simulink model "AutonomousModel_V5"  (R2020b)
settings: Solver=ode23t  StartTime=0.0  StopTime=180.1  FixedStep=0.05  RelTol=1e-3  EnableMultiTasking=on
model workspace (MAT data in the model file):
  DROP_VACCINE_TIME = 0.25
  GRID_SIDE = 0.457142857143
  HALF_TICKS_TO_DIST = 0.00174532925
  LATCHER_OFFSET = 0.3934603175
  LATCH_CELL_TIME = 0.5
  LOWER_PLATFORM_TIME = 0.5
  NUM_SURVEY_GRIDS = 7
  SPACE_SIDE = 0.152380952381
  SURVEY_GRIDS_CELLS = Simulink.Signal
  SURVEY_GRIDS_CELLS.DataType = 'double'
  SURVEY_GRIDS_CELLS.Dimensions = [1 7]
  SURVEY_GRIDS_CELLS.DimensionsMode = 'Fixed'
  SURVEY_GRIDS_CELLS.Complexity = 'real'
  SURVEY_GRIDS_CELLS.SampleTime = -1
  SURVEY_GRIDS_CELLS.SamplingMode = 'auto'
  SURVEY_GRIDS_CELLS.InitialValue = '[3 3 3 3 3 3 3]'
  SURVEY_GRIDS_COORDS = [5  6; 5  5; 5  4; 4  3; 5  2; 5  1; 6  0]
  SURVEY_TURN_ANGLE = 22.7856177106
  WAIT_CONFIRM_CELL_TIME = 0.08
  currentSurveyGridIndex = Simulink.Signal
  currentSurveyGridIndex.DataType = 'double'
  currentSurveyGridIndex.Dimensions = 1
  currentSurveyGridIndex.DimensionsMode = 'Fixed'
  currentSurveyGridIndex.Complexity = 'real'
  currentSurveyGridIndex.SampleTime = -1
  currentSurveyGridIndex.SamplingMode = 'auto'
  currentSurveyGridIndex.InitialValue = '0'
  fullRobotAngle = Simulink.Signal
  fullRobotAngle.DataType = 'double'
  fullRobotAngle.Dimensions = 1
  fullRobotAngle.DimensionsMode = 'Fixed'
  fullRobotAngle.Complexity = 'real'
  fullRobotAngle.SampleTime = -1
  fullRobotAngle.SamplingMode = 'auto'
  fullRobotAngle.InitialValue = '0'
  mapForSim.obsMap = [0 0 0 0 0 0 0 0 0 0 0 0 ... (4194304 elements, 2048x2048)]
  mapForSim.scaleFactor = 409.6
  mapForSim.simMap = robotics.BinaryOccupancyGrid
  mapForSim.simMap.Grid = [1 1 1 1 1 1 1 1 1 1 1 1 ... (4194304 elements, 2048x2048)]
  mapForSim.simMap.LayerName = "binaryLayer"
  mapForSim.simMap.Index = matlabshared.autonomous.internal.CircularBufferIndex
  mapForSim.simMap.Index.Head = [1 1]
  mapForSim.simMap.Index.Size = [2048 2048]
  mapForSim.simMap.Index.NewRegions = [0 0 0 0]
  mapForSim.simMap.Index.DropEntireMap = 0
  mapForSim.simMap.Index.DropTwoRegions = [0 0]
  mapForSim.simMap.Buffer = matlabshared.autonomous.internal.CircularBuffer
  mapForSim.simMap.Buffer.ConstVal = 0
  mapForSim.simMap.Buffer.DataType = 'logical'
  mapForSim.simMap.Buffer.Index = matlabshared.autonomous.internal.CircularBufferIndex
  mapForSim.simMap.Buffer.Index.Head = [1 1]
  mapForSim.simMap.Buffer.Index.Size = [2048 2048]
  mapForSim.simMap.Buffer.Index.NewRegions = [0 0 0 0]
  mapForSim.simMap.Buffer.Index.DropEntireMap = 0
  mapForSim.simMap.Buffer.Index.DropTwoRegions = [0 0]
  mapForSim.simMap.Buffer.Buffer = [1 1 1 1 1 1 1 1 1 1 1 1 ... (4194304 elements, 2048x2048)]
  mapForSim.simMap.DefaultValueInternal = 0
  mapForSim.simMap.HasParent = 0
  mapForSim.simMap.Resolution = 409.6
  mapForSim.simMap.GridSize = [2048 2048]
  mapForSim.simMap.GridOriginInLocal = [0 0]
  mapForSim.simMap.LocalOriginInWorld = [0 0]
  mapForSim.simMap.Width = 5
  mapForSim.simMap.Height = 5
  mapForSim.simMap.LocalOriginInWorldInternal = [0 0]
  moveDir = Simulink.Signal
  moveDir.DataType = 'double'
  moveDir.Dimensions = 1
  moveDir.DimensionsMode = 'Fixed'
  moveDir.Complexity = 'real'
  moveDir.SampleTime = -1
  moveDir.SamplingMode = 'auto'
  moveDir.InitialValue = '0'
  occGrid = robotics.BinaryOccupancyGrid
  occGrid.Grid = [1 1 1 1 1 1 1 1 1 1 1 1 ... (4194304 elements, 2048x2048)]
  occGrid.LayerName = "binaryLayer"
  occGrid.Index = matlabshared.autonomous.internal.CircularBufferIndex
  occGrid.Index.Head = [1 1]
  occGrid.Index.Size = [2048 2048]
  occGrid.Index.NewRegions = [0 0 0 0]
  occGrid.Index.DropEntireMap = 0
  occGrid.Index.DropTwoRegions = [0 0]
  occGrid.Buffer = matlabshared.autonomous.internal.CircularBuffer
  occGrid.Buffer.ConstVal = 0
  occGrid.Buffer.DataType = 'logical'
  occGrid.Buffer.Index = matlabshared.autonomous.internal.CircularBufferIndex
  occGrid.Buffer.Index.Head = [1 1]
  occGrid.Buffer.Index.Size = [2048 2048]
  occGrid.Buffer.Index.NewRegions = [0 0 0 0]
  occGrid.Buffer.Index.DropEntireMap = 0
  occGrid.Buffer.Index.DropTwoRegions = [0 0]
  occGrid.Buffer.Buffer = [1 1 1 1 1 1 1 1 1 1 1 1 ... (4194304 elements, 2048x2048)]
  occGrid.DefaultValueInternal = 0
  occGrid.HasParent = 0
  occGrid.Resolution = 409.6
  occGrid.GridSize = [2048 2048]
  occGrid.GridOriginInLocal = [0 0]
  occGrid.LocalOriginInWorld = [0 0]
  occGrid.Width = 5
  occGrid.Height = 5
  occGrid.LocalOriginInWorldInternal = [0 0]
  oldDetectedCellType = Simulink.Signal
  oldDetectedCellType.DataType = 'double'
  oldDetectedCellType.Dimensions = 1
  oldDetectedCellType.DimensionsMode = 'Fixed'
  oldDetectedCellType.Complexity = 'real'
  oldDetectedCellType.SampleTime = -1
  oldDetectedCellType.SamplingMode = 'auto'
  oldDetectedCellType.InitialValue = 'nan'
  onlyTrackUninfectedCells = Simulink.Signal
  onlyTrackUninfectedCells.DataType = 'boolean'
  onlyTrackUninfectedCells.Dimensions = 1
  onlyTrackUninfectedCells.DimensionsMode = 'Fixed'
  onlyTrackUninfectedCells.Complexity = 'real'
  onlyTrackUninfectedCells.SampleTime = -1
  onlyTrackUninfectedCells.SamplingMode = 'auto'
  onlyTrackUninfectedCells.InitialValue = 'false'
  prevLTicks = Simulink.Signal
  prevLTicks.DataType = 'double'
  prevLTicks.Dimensions = 1
  prevLTicks.DimensionsMode = 'Fixed'
  prevLTicks.Complexity = 'real'
  prevLTicks.SampleTime = -1
  prevLTicks.SamplingMode = 'auto'
  prevLTicks.InitialValue = '0'
  prevRTicks = Simulink.Signal
  prevRTicks.DataType = 'double'
  prevRTicks.Dimensions = 1
  prevRTicks.DimensionsMode = 'Fixed'
  prevRTicks.Complexity = 'real'
  prevRTicks.SampleTime = -1
  prevRTicks.SamplingMode = 'auto'
  prevRTicks.InitialValue = '0'
  straightDistTraveled = Simulink.Signal
  straightDistTraveled.DataType = 'double'
  straightDistTraveled.Dimensions = 1
  straightDistTraveled.DimensionsMode = 'Fixed'
  straightDistTraveled.Complexity = 'real'
  straightDistTraveled.SampleTime = -1
  straightDistTraveled.SamplingMode = 'auto'
  straightDistTraveled.InitialValue = '0'
  unsavedUninfectedCells = Simulink.Signal
  unsavedUninfectedCells.DataType = 'double'
  unsavedUninfectedCells.Dimensions = 1
  unsavedUninfectedCells.DimensionsMode = 'Fixed'
  unsavedUninfectedCells.Complexity = 'real'
  unsavedUninfectedCells.SampleTime = -1
  unsavedUninfectedCells.SamplingMode = 'auto'
  unsavedUninfectedCells.InitialValue = '12'
  xPos = Simulink.Signal
  xPos.DataType = 'double'
  xPos.Dimensions = 1
  xPos.DimensionsMode = 'Fixed'
  xPos.Complexity = 'real'
  xPos.SampleTime = -1
  xPos.SamplingMode = 'auto'
  xPos.InitialValue = '-0.4071428571'
  yPos = Simulink.Signal
  yPos.DataType = 'double'
  yPos.Dimensions = 1
  yPos.DimensionsMode = 'Fixed'
  yPos.Complexity = 'real'
  yPos.SampleTime = -1
  yPos.SamplingMode = 'auto'
  yPos.InitialValue = '1.6'
undefined symbols (not defined in the file): cellLevel, cellPose, cellTypeArray, FloorSurface, isoPoses, platformPoses, PlowSurface, Ref, RobotSurface, WallSurface, X, Y, Z
libraries: sm_lib x286, nesl_utility x157, simulink x72, pid_lib x3
(part 1 of 16)
settings Model: NumberOfSteps=1000  EnablePacing=on  PacingRate=1000  ExtModeTrigDuration=25  OrderedModelArguments=off  Creator=scastro  LastModifiedBy=wanga
settings SolverCC: AlgebraicLoopSolver=LineSearch
settings DataIOCC: LimitDataPoints=on  SignalLogging=off  ReturnWorkspaceOutputs=off
settings OptimizationCC: DefaultParameterBehavior=Inlined  PassReuseOutputArgsAs=Individual arguments  MaxStackSize=64  EfficientTunableParamExpr=on
settings DebuggingCC: ReadBeforeWriteMsg=DisableAll  WriteAfterWriteMsg=DisableAll  WriteAfterReadMsg=DisableAll  MultiTaskDSMMsg=none  ParameterPrecisionLossMsg=none  ParameterTunabilityLossMsg=error  UnconnectedLineMsg=none  AllowSymbolicDim=off  SFUnexpectedBacktrackingDiag=warning  SFNoUnconditionalDefaultTransitionDiag=warning  SFExecutionAtInitializationDiag=none  ArithmeticOperatorsInVariantConditions=warning
settings HardwareCC: ProdBitPerPointer=32  ProdBitPerSizeT=32  ProdBitPerPtrDiffT=32  ProdLargestAtomicInteger=Long  ProdLargestAtomicFloat=Double  ProdWordSize=32  ProdHWDeviceType=ARM Compatible->ARM Cortex
settings ModelReferenceCC: UpdateModelReferenceTargets=IfOutOfDate
settings SFSimCC: SFSimEcho=off  SimUseLocalCustomCode=off  MATLABDynamicMemAlloc=off  CustomCodeUndefinedFunction=UseInterfaceOnly
settings RTWCC: Description=Embedded Coder  SystemTargetFile=ert.tlc  TemplateMakefile=ert_default_tmf  GenerateReport=on  RTWUseLocalCustomCode=off  Toolchain=GNU Tools for ARM Embedded Processors  IncludeHyperlinkInReport=on  LaunchReport=on  GenerateTraceInfo=on  GenerateTraceReport=on  GenerateTraceReportSl=on  GenerateTraceReportSf=on  GenerateTraceReportEml=on
settings CodeAppCC: ForceParamTrailComments=on  IgnoreCustomStorageClasses=off  OperatorAnnotations=on  SimulinkDataObjDesc=on  SFDataObjDesc=on  InsertBlockDesc=on
settings ERTTargetCC: ExtModeStaticAllocSize=2048  ERTCustomFileTemplate=example_file_process.tlc
settings ConfigComp: CovMetricSettings=dw  CovSaveCumulativeToWorkspaceVar=on  CovSaveSingleToWorkspaceVar=on  CovExternalEMLEnable=off  CovSFcnEnable=off
settings SimscapeCC: SimscapeNominalValues="[{\"value\":\"10\",\"unit\":\"V\"},{\"value\":\"1\",\"unit\":\"A\"},{\"value\":\"10\",\"unit\":\"N*m\"},{\"value\":\"10\",\"unit\":\"bar\"},{\"value\":\"100\",\"unit\":\"kJ/kg\"},{\"value\":\"1\",\"unit\":\"kW\"},{\"value\":\"300\",\"unit\":\"K\"},{\"value\":\"100\",\"unit\":\"cm^3/s\"},{\"value\":\"1\",\"unit\":\"kN\"},{\"value\":\"1\",\"unit\":\"g/cm^3\"},{\"value\":\"1\",\"unit\":\"l\"},{\"value\":\"1\",\"unit\":\"cm^2\"},{\"value\":\"60\",\"unit\":\"Hz\"}]"  SimscapeLogOpenViewer=on  SimscapeLogDataHistory=10000
settings ConfigurationSet: Description=SimMechanics 2G
settings DiagnosticsConfigSet: SimMechanicsRigidlyBoundBlock=none
settings ExplorerConfigSet: InternalSimMechanicsExplorerSettings="<ExplorerConfiguration><canonicalview>default</canonicalview><AnimationSetting><BasePlaybackSpeed>1.0</BasePlaybackSpeed><PlaybackSpeedFactor>1.0</PlaybackSpeedFactor></AnimationSetting><TilePanel><TileInfo><Tiles Columns=\"1\" Count=\"1\" Rows=\"1\"><Column Weight=\"1\"/><Row Weight=\"1\"/><Tile Height=\"1\" Width=\"1\" X=\"0\" Y=\"0\"/></Tiles></TileInfo><SceneInfo><SceneViewer><BGColor><R>0.60000002384185791</R><G>0.60000002384185791</G><B>0.60000002384185791</B></BGColor><Camera><DoPerspective>off</DoPerspective><Position><X>0.310056035483453618</X><Y>0.109095541278226044</Y><Z>4.98936036725367327</Z></Position><Center><X>0.310056035483453618</X><Y>0.109095541278226044</Y><Z>-0.0112921193492265814</Z></Center><Up><X>0</X><Y>1</Y><Z>-0</Z></Up><ViewLimDist>1</ViewLimDist><YLim>2.36524049999999963</YLim><XLim>2.81382059482758606</XLim></Camera></SceneViewer></SceneInfo></TilePanel><MechEditorPanel><Cameras><Camera><Id>Camera1</Id><Value><Name>RobotView</Name><NativeCamera><PositionTrackingFeature>BEST_Robotics_2020_Game_Double_Click.BEST_2020_Robot.Body.RobotCamera.F</PositionTrackingFeature><CenterTrackingFeature>BEST_Robotics_2020_Game_Double_Click.BEST_2020_Robot.Body.RobotCamera.F</CenterTrackingFeature><UpVectorTrackingFeature>BEST_Robotics_2020_Game_Double_Click.BEST_2020_Robot.Body.RobotCamera.F</UpVectorTrackingFeature><CenterTrackingOrigin>off</CenterTrackingOrigin><CenterTrackingDirection>+X</CenterTrackingDirection><UpVectorTrackingDirection>+Z</UpVectorTrackingDirection></NativeCamera></Value></Camera></Cameras><GfxPanelCameraMap/><VideoCreator><PlaybackSpeedRatio>1.0</PlaybackSpeedRatio><FrameRate>16</FrameRate><VideoFormat>Motion JPEG AVI</VideoFormat><FrameSize>auto</FrameSize></VideoCreator></MechEditorPanel></ExplorerConfiguration>"

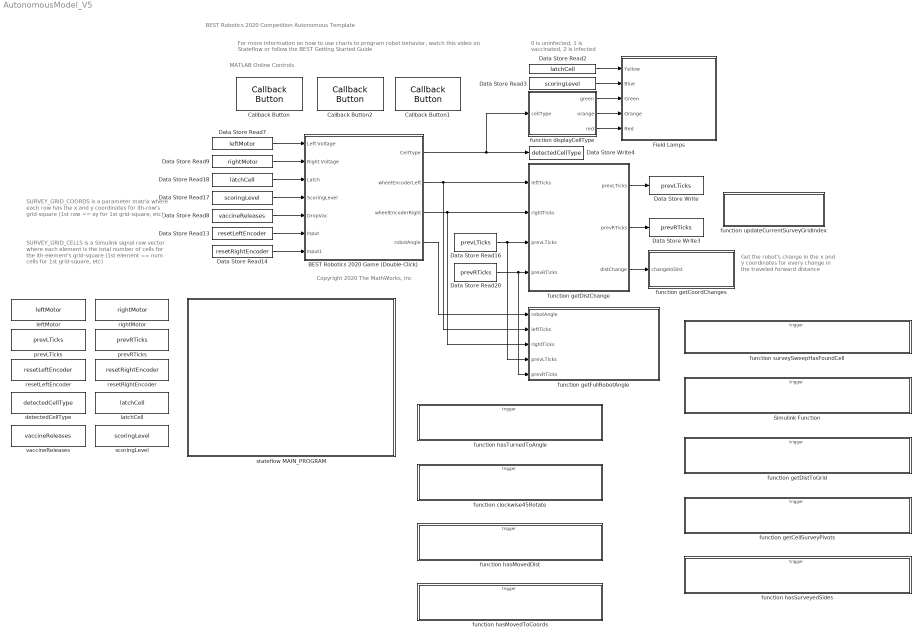
== system AutonomousModel_V5 ==
  note: 0 is uninfected, 1 is vaccinated, 2 is infected
  note: SURVEY_GRID_CELLS is a Simulink signal row vector where each element is the total number of cells for the ith-element's grid-square (1st element == num cells for 1st grid-square, etc)
  note: SURVEY_GRID_COORDS is a parameter matrix where each row has the x and y coordinates for ith-row's grid-square (1st row == xy for 1st grid-square, etc)
  note: MATLAB Online Controls
  note: For more information on how to use charts to program robot behavior,
      | watch this video on Stateflow or follow the BEST Getting Started Guide
  note: BEST Robotics 2020 Competition Autonomous Template
  note: Copyright 2020 The MathWorks, Inc
  note: Get the robot's change in the x and y coordinates for
      | every change in the traveled forward distance
  BEST Robotics 2020 Game (Double-Click) : Subsystem  mask(RP BEST Robotics 2020 Challenge){gameTime=180, field=Practice 2, rvis=off, sensor=off, autoField=on, wheelBase=0.5, wheelRadius=0.1, robotColor=[0.5 0 0], wheelThickness=0.025, chassisThickness=0.05, wheelMass=1, chassisMass=1.5}
      mask prompts: gameTime "Game Time (s)"; field "Field Layout"; rvis "Show cell type after run (Runs slower)"; sensor "Activate Gripper Sensor (Not allowed during competition)"; autoField "Autonomous Configuration"; wheelBase "Distance between wheels [m]"; wheelRadius "Wheel radius [m]"; robotColor "Color [R G B]"; wheelThickness "Wheel Thickness [m]"; chassisThickness "Chassis Thickness [m]"; wheelMass "Wheel Mass [kg]"; chassisMass "Chassis Mass [kg]"
      mask help:
      | This block contains a virtual game for the BEST Robotics 2020 competition. Please refere to the instructions provided by competition organizers for more information on game rules.
      |
      | Inputs:
      | Motor Voltages (Torque) [-127 to 127]
      | LatchCell (Pickup Cell) [0 or 1]
      | ScoringLevel (Floor or Platform) [0 or 1]
      | DropVac (Release vaccine) [0 or 1] Array of 3
      |
      | Outputs:
      | Cell Type (Uninfected, Immune, Infected) [0 ,1 or 2]
      | Sensors (See inside block for sensor properties and outputs)
      |
      | For MATLAB and Simulink related questions please email: roboticsarena@mathworks.com
      mask init:
      | autochoice=get_param(gcb,'autoField');
      | choice=get_param(gcb,'field');
      | time=get_param(gcb,'gameTime');
      | set_param(gcs,'StopTime',num2str(str2num(time)+0.1));
      | 
      | if strcmp(choice,'Practice 1')
      |   BEST2020GameConfig1 
      | elseif strcmp(choice,'Practice 2')
      |   BEST2020GameConfig2 
      | elseif strcmp(choice,'Practice 3')
      |   BEST2020GameConfig3 
      | elseif strcmp(choice,'Random')
      |   BEST2020GameConfigRand
      | elseif strcmp(autochoice,"on")
      |    if strcmp(choice,'Competition 1 (Provided during competition)')
      |      BEST2020GameConfigAuto1
      |    elseif strcmp(choice,'Competition 2 (Provided during competition)')
      |      BEST2020GameConfigAuto2
      |    elseif strcmp(choice,'Competition 3 (Provided during competition)')
      |      BEST2020GameConfigAuto3
      |    elseif strcmp(choice,'Competition 4 (Provided during competition)')
      |      BEST2020GameConfigAuto4
      |    elseif strcmp(choice,'Competition 5 (Provided during competition)')
      |      BEST2020GameConfigAuto5
      |    elseif strcmp(choice,'Competition 6 (Provided during competition)')
      |      BEST2020GameConfigAuto6
      |    elseif strcmp(choice,'Competition 7 (Provided during competition)')
      |      BEST2020GameConfigAuto7
      |    elseif strcmp(choice,'Competition 8 (Provided during competition)')
      |      BEST2020GameConfigAuto8
      |    else
      |      BEST2020GameConfigAuto1
      |    end
      | elseif strcmp(choice,'Competition 1 (Provided during competition)')
      |   BEST2020GameConfigComp1
      | elseif strcmp(choice,'Competition 2 (Provided during competition)')
      |   BEST2020GameConfigComp2
      | elseif strcmp(choice,'Competition 3 (Provided during competition)')
      |   BEST2020GameConfigComp3
      | elseif strcmp(choice,'Competition 4 (Provided during competition)')
      |   BEST2020GameConfigComp4
      | elseif strcmp(choice,'Competition 5 (Provided during competition)')
      |   BEST2020GameConfigComp5
      | elseif strcmp(choice,'Competition 6 (Provided during competition)')
      |   BEST2020GameConfigComp6
      | elseif strcmp(choice,'Competition 7 (Provided during competition)')
      |   BEST2020GameConfigComp7
      | elseif strcmp(choice,'Competition 8 (Provided during competition)')
      |   BEST2020GameConfigComp8
      | else
      |   BEST2020GameConfig1 
      | end
      mask TypeOptions field: Practice 1 | Practice 2 | Practice 3 | Random | Competition 1 (Provided during competition) | Competition 2 (Provided during competition) | Competition 3 (Provided during competition) | Competition 4 (Provided during competition) | Competition 5 (Provided during competition) | Competition 6 (Provided during competition) | Competition 7 (Provided during competition) | Competition 8 (Provided during competition)
      mask Callback rvis:
      | visual=get_param(gcb,'rvis');
      | for i=1:21
      |     if strcmp(visual,'off')
      |         set_param([gcb '/Cells/Object' num2str(i) '/EndVisuals'],'Commented','on');
      |     else
      |         set_param([gcb '/Cells/Object' num2str(i) '/EndVisuals'],'Commented','off');
      |     end
      | end
      mask TypeOptions wheelThickness: BEST 2020 Robot/wheelThickness
      mask TypeOptions chassisThickness: BEST 2020 Robot/chassisThickness
      mask TypeOptions wheelMass: BEST 2020 Robot/wheelMass
      mask TypeOptions chassisMass: BEST 2020 Robot/chassisMass
      mask DialogControl Container8 Prompt: Game Settings
      mask DialogControl Container4 Prompt: Robot settings
      mask Display:
      | image('BEST2020Environment.png')
      | port_label('input',1,'LeftMotor')
      | port_label('input',2,'RightMotor')
      | port_label('input',3,'LatchCell')
      | port_label('input',4,'ScoringLevel')
      | port_label('input',5,'DropVac')
      | port_label('output',1,'CellType')
      | port_label('output',2,'LeftEncoder')
      | port_label('output',3,'RightEncoder')
      | port_label('output',4,'RobotAngle')
  Callback Button : CallbackButton  ButtonText=Create Simulation Video (FPV)
      settings: ClickFcn=|
      | %% Simulate Model and Create Video
      | model=gcs;
      | disp(['Simulating Model: ' model '...'])
      | w=waitbar(0,['Simulating Model: ' model '...']);
      | set_param(model, 'EnablePacing', 'off');
      | sim(model);
      | set_param(model, 'EnablePacing', 'on');
      | disp('Creating Simulation Video...')
      | waitbar(0.5,w,'Creating Simulation Video...')
      | smwritevideo(model,model,'FrameRate',16,'FrameSize',[1280 720],'Tile',1)
      | disp('Animation window will close when completed')
      | waitbar(1,w,'Animation window will close when completed')
      | pause(5)
      | close(w)
  Callback Button1 : CallbackButton  ButtonText=Re-play Simulation Video
      settings: ClickFcn=|
      | %% Playback Simulation Video
      | disp('Replaying Simulation Video...')
      | videoReader = VideoReader([gcs '.avi']);
      | videoPlayer = vision.VideoPlayer('Position',[100 100 1280 720]);
      | 
      | % Play video. Every call to the step method reads another frame.
      | 
      | while hasFrame(videoReader)
      |    frame = readFrame(videoReader);
      |    step(videoPlayer,frame);
      |    pause(1/16);
      | end
      | disp('Done replaying simulation video')
  Callback Button2 : CallbackButton  ButtonText=Create Simulation Video (Top View)
      settings: ClickFcn=|
      | %% Simulate Model and Create Video
      | model=gcs;
      | disp(['Simulating Model: ' model '...'])
      | w=waitbar(0,['Simulating Model: ' model '...']);
      | set_param(model, 'EnablePacing', 'off');
      | sim(model);
      | set_param(model, 'EnablePacing', 'on');
      | disp('Creating Simulation Video...')
      | waitbar(0.5,w,'Creating Simulation Video...')
      | smwritevideo(model,model,'FrameRate',16,'FrameSize',[1280 720],'Tile',3)
      | disp('Animation window will close when completed')
      | waitbar(1,w,'Animation window will close when completed')
      | pause(5)
      | close(w)
  Data Store Read13 : DataStoreRead  DataStoreName=resetLeftEncoder
  Data Store Read14 : DataStoreRead  DataStoreName=resetRightEncoder
  Data Store Read16 : DataStoreRead  DataStoreName=prevLTicks
  Data Store Read17 : DataStoreRead  DataStoreName=scoringLevel
  Data Store Read18 : DataStoreRead  DataStoreName=latchCell
  Data Store Read2 : DataStoreRead  DataStoreName=latchCell
  Data Store Read20 : DataStoreRead  DataStoreName=prevRTicks
  Data Store Read3 : DataStoreRead  DataStoreName=scoringLevel
  Data Store Read7 : DataStoreRead  DataStoreName=leftMotor
  Data Store Read8 : DataStoreRead  DataStoreName=vaccineReleases
  Data Store Read9 : DataStoreRead  DataStoreName=rightMotor
  Data Store Write : DataStoreWrite  DataStoreName=prevLTicks
  Data Store Write3 : DataStoreWrite  DataStoreName=prevRTicks
  Data Store Write4 : DataStoreWrite  DataStoreName=detectedCellType
  Field Lamps : Subsystem
      mask Display:
      | image('lamps.PNG')
      | port_label('input',1,'Yellow')
      | port_label('input',2,'Blue')
      | port_label('input',3,'Green')
      | port_label('input',4,'Orange')
      | port_label('input',5,'Red')
  Simulink Function : Subsystem  TreatAsAtomicUnit=on
  detectedCellType : DataStoreMemory  DataStoreName=detectedCellType  ReadBeforeWriteMsg=warning  WriteAfterWriteMsg=warning  WriteAfterReadMsg=warning  ShowAdditionalParam=off  OutDataTypeStr=double  Dimensions=1
  function clockwise45Rotate : Subsystem  TreatAsAtomicUnit=on
  function displayCellType : MATLAB Function  TreatAsAtomicUnit=on
  function getCellSurveyPivots : Subsystem  TreatAsAtomicUnit=on
  function getCoordChanges : MATLAB Function  TreatAsAtomicUnit=on
  function getDistChange : MATLAB Function  TreatAsAtomicUnit=on
  function getDistToGrid : Subsystem  TreatAsAtomicUnit=on
  function getFullRobotAngle : MATLAB Function  TreatAsAtomicUnit=on
  function hasMovedDist : Subsystem  TreatAsAtomicUnit=on
  function hasMovedToCoords : Subsystem  TreatAsAtomicUnit=on
  function hasSurveyedSides : Subsystem  TreatAsAtomicUnit=on
  function hasTurnedToAngle : Subsystem  TreatAsAtomicUnit=on
  function surveySweepHasFoundCell : Subsystem  TreatAsAtomicUnit=on
  function updateCurrentSurveyGridIndex : MATLAB Function  TreatAsAtomicUnit=on
  latchCell : DataStoreMemory  DataStoreName=latchCell  ReadBeforeWriteMsg=warning  WriteAfterWriteMsg=warning  WriteAfterReadMsg=warning  ShowAdditionalParam=off  OutDataTypeStr=double  Dimensions=1
  leftMotor : DataStoreMemory  DataStoreName=leftMotor  ReadBeforeWriteMsg=warning  WriteAfterWriteMsg=warning  WriteAfterReadMsg=warning  ShowAdditionalParam=off  OutDataTypeStr=double  Dimensions=1
  prevLTicks : DataStoreMemory  DataStoreName=prevLTicks  ReadBeforeWriteMsg=warning  WriteAfterWriteMsg=warning  WriteAfterReadMsg=warning  ShowAdditionalParam=off  OutDataTypeStr=double  Dimensions=1
  prevRTicks : DataStoreMemory  DataStoreName=prevRTicks  ReadBeforeWriteMsg=warning  WriteAfterWriteMsg=warning  WriteAfterReadMsg=warning  ShowAdditionalParam=off  OutDataTypeStr=double  Dimensions=1
  resetLeftEncoder : DataStoreMemory  DataStoreName=resetLeftEncoder  ReadBeforeWriteMsg=warning  WriteAfterWriteMsg=warning  WriteAfterReadMsg=warning  ShowAdditionalParam=off  OutDataTypeStr=double  Dimensions=1
  resetRightEncoder : DataStoreMemory  DataStoreName=resetRightEncoder  ReadBeforeWriteMsg=warning  WriteAfterWriteMsg=warning  WriteAfterReadMsg=warning  ShowAdditionalParam=off  OutDataTypeStr=double  Dimensions=1
  rightMotor : DataStoreMemory  DataStoreName=rightMotor  ReadBeforeWriteMsg=warning  WriteAfterWriteMsg=warning  WriteAfterReadMsg=warning  ShowAdditionalParam=off  OutDataTypeStr=double  Dimensions=1
  scoringLevel : DataStoreMemory  DataStoreName=scoringLevel  ReadBeforeWriteMsg=warning  WriteAfterWriteMsg=warning  WriteAfterReadMsg=warning  ShowAdditionalParam=off  OutDataTypeStr=double  Dimensions=1
  stateflow MAIN_PROGRAM : Stateflow chart  TreatAsAtomicUnit=on
  vaccineReleases : DataStoreMemory  DataStoreName=vaccineReleases  ReadBeforeWriteMsg=warning  WriteAfterWriteMsg=warning  WriteAfterReadMsg=warning  InitialValue=[0 0 0]  VectorParams1D=off  ShowAdditionalParam=off  OutDataTypeStr=fixdt('double', 'DataTypeOverride', 'Off')  Dimensions=[1 3]
      settings: LockScale=on
  wires:
  Data Store Read9/1 -> BEST Robotics 2020 Game (Double-Click)/2(Right Voltage)
  BEST Robotics 2020 Game (Double-Click)/1(CellType) -> function displayCellType/1(cellType), Data Store Write4/1
  function displayCellType/1(green) -> Field Lamps/3(Green)
  function displayCellType/3(red) -> Field Lamps/5(Red)
  function displayCellType/2(orange) -> Field Lamps/4(Orange)
  Data Store Read8/1 -> BEST Robotics 2020 Game (Double-Click)/5(DropVac)
  Data Store Read7/1 -> BEST Robotics 2020 Game (Double-Click)/1(Left Voltage)
  Data Store Read13/1 -> BEST Robotics 2020 Game (Double-Click)/6(Input)
  Data Store Read14/1 -> BEST Robotics 2020 Game (Double-Click)/7(Input1)
  BEST Robotics 2020 Game (Double-Click)/3(wheelEncoderRight) -> function getFullRobotAngle/3(rightTicks), function getDistChange/2(rightTicks)
  Data Store Read20/1 -> function getFullRobotAngle/5(prevRTicks), function getDistChange/4("prevRTicks ")
  function getDistChange/3(distChange) -> function getCoordChanges/1(changeInDist)
  Data Store Read16/1 -> function getFullRobotAngle/4(prevLTicks), function getDistChange/3("prevLTicks ")
  BEST Robotics 2020 Game (Double-Click)/2(wheelEncoderLeft) -> function getFullRobotAngle/2(leftTicks), function getDistChange/1(leftTicks)
  BEST Robotics 2020 Game (Double-Click)/4(robotAngle) -> function getFullRobotAngle/1(robotAngle)
  Data Store Read17/1 -> BEST Robotics 2020 Game (Double-Click)/4(ScoringLevel)
  Data Store Read18/1 -> BEST Robotics 2020 Game (Double-Click)/3(Latch)
  Data Store Read3/1 -> Field Lamps/2(Blue)
  Data Store Read2/1 -> Field Lamps/1(Yellow)
  function getDistChange/1(prevLTicks) -> Data Store Write/1
  function getDistChange/2(prevRTicks) -> Data Store Write3/1

== system AutonomousModel_V5/BEST Robotics 2020 Game (Double-Click) ==
  note: DO NOT CHANGE THIS MODEL!
  Left Voltage : Inport
  Right Voltage : Inport  Port=2
  Latch : Inport  Port=3
  ScoringLevel : Inport  Port=4
  DropVac : Inport  Port=5
  Input : Inport  Port=6
  Input1 : Inport  Port=7
  Arena : Subsystem  mask(RP Grid Arena){length=7, width=7}
      mask prompts: length "Arena length [m]"; width "Arena width [m]"
      mask help: This block is an arena for robots to operate within. This arena implements contact between one robot and the walls and also introduces a floor grid for better visualization. Connect to other robots within the library using the corresponding "Robot" and "Ref" ports.
      mask DialogControl Container5 Prompt: Arena dimensions
      mask Display:
      | image('BEST2020Arena.png')
      | port_label('Lconn',1,'RP-Bus')
  BEST 2020 Robot : Subsystem  mask(RP Contact Tank Robot){robotId=1, wheelRadius=wheelRadius, wheelBase=wheelBase, wheelThickness=wheelThickness, chassisThickness=chassisThickness, startPose=[-2 0], choice=off, sensorTs=0.05, wheelMass=wheelMass, chassisMass=chassisMass, maxWheelTorque=2, wheelColor=[0.25 0.25 0.25], chassisColor=robotColor}
      mask prompts: robotId "Robot ID"; wheelRadius "Wheel Radius [m]"; wheelBase "Wheelbase [m]"; wheelThickness "Wheel Thickness [m]"; chassisThickness "Chassis Thickness [m]"; startPose "Start Position [m]"; choice "Reverse Start Position"; sensorTs "Sensor sample time [s]"; wheelMass "Wheel Mass [kg]"; chassisMass "Chassis Mass [kg]"; maxWheelTorque "Maximum wheel torque [N*m]"; wheelColor "Wheel Color"; chassisColor "Chassis Color"
      mask help:
      | This robot implements contact between the robot wheels and the floor of an arena. The stck-slip friction implemented using contact force libraries makes the robot behavior more realistic. The inputs to the robot are now motor torque, which is set using the Robotics Playground Motor blocks. The motor mappings are as follows:
      |
      | Motor 1 -> Left wheel motor torque
      | Motor 2 -> Right wheel motor torque
      mask DialogControl KinContainer Prompt: Kinematics
      mask DialogControl DynamicsContainer Prompt: Dynamics
      mask DialogControl AppearanceContainer Prompt: Appearance
      mask Display:
      | image('BEST2020Robot.png')
      | port_label('Rconn',1,'RP-Bus')
  Cells : Subsystem
      mask Display: image('BEST2020Cells.png')
  Compass Sensor : Subsystem  mask(RP Compass Sensor){sensorTs=.1}
      mask prompts: sensorTs "Sensor sample time [s]"
      mask help: This sensor outputs the rotation in degrees as measured from the robot center relative to the world coordinate frame.
      mask Help: web('compass_sensor.htm')
      mask DialogControl senCont Prompt: Sensor Characteristics
      mask Display:
      | color('white');
      | plot([100,100,100,100]*1,[100,100,100,100]*1);
      | plot([100,100,100,100]*0,[100,100,100,100]*0);
      | image('Compass.png','center')
      | color('blue');
  Game Control : Subsystem
  Left Encoder1 : Subsystem  mask(RP Motor Encoder){rstChoice=Reset by external signal, ticks=180, detectDir=on, sensorTs=.1}
      mask prompts: rstChoice "Reset option"; ticks "Ticks per rotation"; detectDir "Detect direction of rotation"; sensorTs "Sensor sample time [s]"
      mask help:
      | This block outputs the rotation in tick counts of an encoder conneted to the respective robot motor. You can set different sensor parameters from the mask or use the default settings.
      |
      | The most common use of motor encoders is to derive the position of an object. Start by converting the tick counts to revolutions of the motor shaft. You can later relate the revolutions of the motor shaft to more valuable robot information such as traveled distance by using robot dimensions like the wheel size.
      mask Help: web('encoder_sensor.htm')
      mask TypeOptions rstChoice: No reset | Reset by external signal
      mask DialogControl ParameterGroupVar Prompt: Settings
      mask Display:
      | color('white');
      | plot([100,100,100,100]*1,[100,100,100,100]*1);
      | plot([100,100,100,100]*0,[100,100,100,100]*0);
      | image('encoder.jpg','center')
  Right Encoder1 : Subsystem  mask(RP Motor Encoder){rstChoice=Reset by external signal, ticks=180, detectDir=on, sensorTs=.1}
      mask prompts: rstChoice "Reset option"; ticks "Ticks per rotation"; detectDir "Detect direction of rotation"; sensorTs "Sensor sample time [s]"
      mask help:
      | This block outputs the rotation in tick counts of an encoder conneted to the respective robot motor. You can set different sensor parameters from the mask or use the default settings.
      |
      | The most common use of motor encoders is to derive the position of an object. Start by converting the tick counts to revolutions of the motor shaft. You can later relate the revolutions of the motor shaft to more valuable robot information such as traveled distance by using robot dimensions like the wheel size.
      mask Help: web('encoder_sensor.htm')
      mask TypeOptions rstChoice: No reset | Reset by external signal
      mask DialogControl ParameterGroupVar Prompt: Settings
      mask Display:
      | color('white');
      | plot([100,100,100,100]*1,[100,100,100,100]*1);
      | plot([100,100,100,100]*0,[100,100,100,100]*0);
      | image('encoder.jpg','center')
  Vaccines : Subsystem
      mask Display: image('BEST2020Vaccines.png')
  CellType : Outport
  wheelEncoderLeft : Outport  Port=2
  wheelEncoderRight : Outport  Port=3
  robotAngle : Outport  Port=4
  wires:
  Right Voltage/1 -> BEST 2020 Robot/2(In2)
  Left Voltage/1 -> BEST 2020 Robot/1(In1)
  Latch/1 -> Cells/1(Latch)
  Cells/1(CellType) -> CellType/1
  Right Encoder1/1(Out1) -> wheelEncoderRight/1
  Left Encoder1/1(Out1) -> wheelEncoderLeft/1
  BEST 2020 Robot/3(angle) -> Compass Sensor/1(angle)
  Compass Sensor/1(Distance) -> robotAngle/1
  DropVac/1 -> Vaccines/2(Drop)
  ScoringLevel/1 -> Vaccines/1("ScoreLevel "), Cells/2(ScoringLevel)
  BEST 2020 Robot/1(leftMotorW) -> Left Encoder1/1(In1)
  BEST 2020 Robot/2(rightMotorW) -> Right Encoder1/1(In1)
  Input/1 -> Left Encoder1/2(Input)
  Input1/1 -> Right Encoder1/2(Input)
  connections:
  Vaccines/LConn1 -- Arena/LConn1 -- BEST 2020 Robot/RConn1 -- Cells/LConn1

== system AutonomousModel_V5/Field Lamps ==
  note: DO NOT EDIT
  note: Inputs should be 0 or 1
  Yellow : Inport
  Blue : Inport  Port=2
  Green : Inport  Port=3
  Orange : Inport  Port=4
  Red : Inport  Port=5
  tag scope: blueLamp=global, greenLamp=global, orangeLamp=global, redLamp=global, yellowLamp=global
  wires:
  Yellow/1 -> [yellowLamp]
  Blue/1 -> [blueLamp]
  Orange/1 -> [orangeLamp]
  Red/1 -> [redLamp]
  Green/1 -> [greenLamp]

== system AutonomousModel_V5/Simulink Function ==
  getNearestUnrescuedGrid : TriggerPort  TriggerType=function-call  IsSimulinkFunction=on  FunctionName=getNearestUnrescuedGrid  FunctionVisibility=scoped  VariantControl=(inherit)
  function getClosestValidGrid : MATLAB Function  TreatAsAtomicUnit=on
  rescueGridX : ArgOut  DisableCoverage=on  ArgumentName=rescueGridX
  rescueGridY : ArgOut  DisableCoverage=on  Port=2  ArgumentName=rescueGridY
  closestGridIndex : ArgOut  DisableCoverage=on  Port=3  ArgumentName=closestGridIndex
  wires:
  function getClosestValidGrid/1(closestGridX) -> rescueGridX/1
  function getClosestValidGrid/2(closestGridY) -> rescueGridY/1
  function getClosestValidGrid/3(closestGridIndex) -> closestGridIndex/1

== system AutonomousModel_V5/function clockwise45Rotate ==
  clockwise45Rotate : TriggerPort  TriggerType=function-call  IsSimulinkFunction=on  FunctionName=clockwise45Rotate  FunctionVisibility=scoped  VariantControl=(inherit)
  function clockwise45Rotate : MATLAB Function  TreatAsAtomicUnit=on
  oldX : ArgIn  DisableCoverage=on  ArgumentName=oldX
  oldY : ArgIn  Port=2  ArgumentName=oldY
  rotatedX : ArgOut  DisableCoverage=on  ArgumentName=rotatedX
  rotatedY : ArgOut  Port=2  ArgumentName=rotatedY
  wires:
  oldX/1 -> function clockwise45Rotate/1(oldX)
  oldY/1 -> function clockwise45Rotate/2(oldY)
  function clockwise45Rotate/1(rotatedX) -> rotatedX/1
  function clockwise45Rotate/2(rotatedY) -> rotatedY/1

== system AutonomousModel_V5/function getCellSurveyPivots ==
  getCellSurveyPivots : TriggerPort  TriggerType=function-call  IsSimulinkFunction=on  FunctionName=getCellSurveyPivots  FunctionVisibility=scoped  VariantControl=(inherit)
  function getCellSurveyCheckpoints : MATLAB Function  TreatAsAtomicUnit=on
  gridX : ArgIn  DisableCoverage=on  ArgumentName=gridX
  gridY : ArgIn  Port=2  ArgumentName=gridY
  pivotSide : ArgOut  DisableCoverage=on  PortDimensions=[1 1]  ArgumentName=pivotSide
  startPivotPoint : ArgOut  Port=2  PortDimensions=[1 2]  ArgumentName=startPivotPoint
  finalPoint : ArgOut  Port=3  PortDimensions=[1 2]  ArgumentName=finalPoint
  wires:
  gridX/1 -> function getCellSurveyCheckpoints/1(gridX)
  gridY/1 -> function getCellSurveyCheckpoints/2(gridY)
  function getCellSurveyCheckpoints/1(pivotSide) -> pivotSide/1
  function getCellSurveyCheckpoints/2(startPivotPoint) -> startPivotPoint/1
  function getCellSurveyCheckpoints/3(finalPoint) -> finalPoint/1

== system AutonomousModel_V5/function getDistToGrid ==
  getDistToGrid : TriggerPort  TriggerType=function-call  IsSimulinkFunction=on  FunctionName=getDistToGrid  FunctionVisibility=scoped  VariantControl=(inherit)
  MATLAB Function : MATLAB Function  TreatAsAtomicUnit=on
  gridX : ArgIn  DisableCoverage=on  ArgumentName=gridX
  gridY : ArgIn  DisableCoverage=on  Port=2  ArgumentName=gridY
  dist : ArgOut  DisableCoverage=on  ArgumentName=dist
  wires:
  MATLAB Function/1(dist) -> dist/1
  gridX/1 -> MATLAB Function/1(gridX)
  gridY/1 -> MATLAB Function/2(gridY)

== system AutonomousModel_V5/function hasMovedDist ==
  note: PID_SETTLE_TIME is measured in n*0.1 seconds,
      | meaning a value of 5 for this would mean a
      | requirement for the PID to turn the robot should
      | settle for 0.5 seconds before stopping
  hasMovedDist : TriggerPort  TriggerType=function-call  IsSimulinkFunction=on  FunctionName=hasMovedDist  FunctionVisibility=scoped  VariantControl=(inherit)
  Abs1 : Abs
  Data Store Memory2 : DataStoreMemory  DataStoreName=settledTime  ReadBeforeWriteMsg=warning  WriteAfterWriteMsg=warning  WriteAfterReadMsg=warning  ShowAdditionalParam=off  OutDataTypeStr=double  Dimensions=1
  Data Store Read6 : DataStoreRead  DataStoreName=settledTime
  Data Store Write1 : DataStoreWrite  DataStoreName=leftMotor
  Data Store Write2 : DataStoreWrite  DataStoreName=rightMotor
  GreaterThanOrEqual1 : RelationalOperator  OutDataTypeStr=boolean  RndMeth=Simplest
  PID Controller : pid_lib/PID Controller  Controller=P  Form=Parallel  TimeDomain=Discrete-time  UseExternalTs=on  SampleTime=0.1  IntegratorMethod=Forward Euler  FilterMethod=Forward Euler  ControllerParametersSource=internal  P=100  I=2  D=0.5  UseFilter=on  N=100  TunerSelectOption=Transfer Function Based (PID Tuner App)  InitialConditionSource=internal  InitialConditionForIntegrator=0  InitialConditionForFilter=0  DifferentiatorICPrevScaledInput=0  ExternalReset=none  TrackingMode=off  Kt=1  LimitOutput=on  SatLimitsSource=internal  UpperSaturationLimit=127  LowerSaturationLimit=-127  LinearizeAsGain=off  AntiWindupMode=none  Kb=1  RndMeth=Nearest  POutMin=[]  POutMax=[]  IOutMin=[]  IOutMax=[]  DOutMin=[]  DOutMax=[]  NOutMin=[]  NOutMax=[]  SumOutMin=[]  SumOutMax=[]  SaturationOutMin=[]  SaturationOutMax=[]  PParamMin=[]  PParamMax=[]  IParamMin=[]  IParamMax=[]  DParamMin=[]  DParamMax=[]  NParamMin=[]  NParamMax=[]  KbParamMin=[]  KbParamMax=[]  KtParamMin=[]  KtParamMax=[]  KbOutMin=[]  KbOutMax=[]  KtOutMin=[]  KtOutMax=[]  IntegratorOutMin=[]  IntegratorOutMax=[]  FilterOutMin=[]  FilterOutMax=[]  SumI1OutMin=[]  SumI1OutMax=[]  SumI2OutMin=[]  SumI2OutMax=[]  SumI3OutMin=[]  SumI3OutMax=[]  SumI4OutMin=[]  SumI4OutMax=[]  SumDOutMin=[]  SumDOutMax=[]  DifferentiatorOutMin=[]  DifferentiatorOutMax=[]  FilterDiffOutCoefMin=[]  FilterDiffOutCoefMax=[]  ReciprocalOutMin=[]  ReciprocalOutMax=[]  SumDenOutMin=[]  SumDenOutMax=[]  SumNumOutMin=[]  SumNumOutMax=[]  DivideOutMin=[]  DivideOutMax=[]  UdiffTsProdOutMin=[]  UdiffTsProdOutMax=[]  NTsProdOutMin=[]  NTsProdOutMax=[]  UintegralTsProdOutMin=[]  UintegralTsProdOutMax=[]  UngainTsProdOutMin=[]  UngainTsProdOutMax=[]  IntegratorContinuousStateAttributes=''  IntegratorStateMustResolveToSignalObject=off  IntegratorRTWStateStorageClass=Auto  FilterContinuousStateAttributes=''  FilterStateMustResolveToSignalObject=off  FilterRTWStateStorageClass=Auto  ParallelPVariant=InternalParameters  IdealPVariant=Disabled  IVariant=Disabled  DVariant=Disabled  IntegratorVariant=Disabled  SatVariant=Enabled  AWVariant=Disabled  PCopyVariant=Disabled  TRVariant=Disabled  FdbkBlocksVariant=Forward  IdealPFdbkVariant=Disabled  SatFdbkVariant=Disabled  DerivativeFilterVariant=Disabled  NVariant=Disabled  NCopyVariant=Disabled_SignalSpec  FilterICVariant=Disabled  IntegratorICVariant=Disabled  ExternalResetVariant=Disabled  TRSumVariant=Passthrough  SumFdbkVariant=Disabled  SumVariant=Passthrough_P  TsampFilterVariant=InternalTs  TsampNgainVariant=Passthrough  TsampIntegralVariant=Disabled  ExternalSaturationOutDataTypeStr=Inherit: Same as second input
  PID_DIST_TOLERANCE : Constant  Value=0.009
  PID_SETTLE_TIME : Constant  Value=2
  function getErrorDist : MATLAB Function  TreatAsAtomicUnit=on
  function getMoveDirSign : MATLAB Function  TreatAsAtomicUnit=on
  stateflow integrateSettleTime : Stateflow chart  TreatAsAtomicUnit=on
      settings: PortSchema="{\"entries\":[{\"content\":{\"sides\":[{\"content\":{\"connectorIds\":[\"In2\",\"In1\"]},\"type\":\"ConnectorPlacement.EquallySpacedRectSide\",\"uuid\":\"f923337d-3128-4ed8-bb4f-3ea7b5686e2d\"},{\"content\":{\"connectorIds\":[],\"side\":\"RIGHT\"},\"type\":\"ConnectorPlacement.EquallySpacedRectSide\",\"uuid\":\"39dc7172-a5aa-4f5c-b2a4-4c61f2fa72eb\"},{\"content\":{\"connectorIds\":[],\"side\":\"TOP\"},\"type\":\"ConnectorPlacement.EquallySpacedRectSide\",\"uuid\":\"39425eec-6ca1-4a0a-a982-d9b02b3e3e8f\"},{\"content\":{\"connectorIds\":[],\"side\":\"HIDDEN\"},\"type\":\"ConnectorPlacement.EquallySpacedRectSide\",\"uuid\":\"aee45ecb-1b8b-4c38-bfd6-fdbe8fac54d7\"}]},\"type\":\"ConnectorPlacement.EquallySpacedConnector\",\"uuid\":\"e05cbbda-f452-42ce-8e08-9c45c77a95c5\"}],\"packageUris\":[\"http://schema.mathworks.com/mf0/Connector/R2020b\"],\"version\":\"1.0\"}"
  stateflow postSettleDist : Stateflow chart  TreatAsAtomicUnit=on
  targetDist : ArgIn  DisableCoverage=on  ArgumentName=targetDist
  distHasSettled : ArgOut  DisableCoverage=on  OutDataTypeStr=boolean  ArgumentName=distHasSettled
  wires:
  GreaterThanOrEqual1/1 -> stateflow postSettleDist/1(distHasSettled), distHasSettled/1
  PID_SETTLE_TIME/1 -> GreaterThanOrEqual1/2
  PID_DIST_TOLERANCE/1 -> stateflow integrateSettleTime/1(TOLERANCE)
  Abs1/1 -> stateflow integrateSettleTime/2(error)
  Data Store Read6/1 -> GreaterThanOrEqual1/1
  function getErrorDist/1(errorDist) -> Abs1/1, PID Controller/1
  targetDist/1 -> function getErrorDist/1(targetDist)
  PID Controller/1 -> Data Store Write2/1, Data Store Write1/1, function getMoveDirSign/1(u)

== system AutonomousModel_V5/function hasMovedToCoords ==
  hasMovedToCoords : TriggerPort  TriggerType=function-call  IsSimulinkFunction=on  FunctionName=hasMovedToCoords  FunctionVisibility=scoped  VariantControl=(inherit)
  stateflow hasMovedToCoords : Stateflow chart  AncestorBlock=RoboticsPlayground/Utilities and Hardware/Stateflow  TreatAsAtomicUnit=on
  xCoord : ArgIn  DisableCoverage=on  ArgumentName=xCoord
  yCoord : ArgIn  Port=2  ArgumentName=yCoord
  useRobotPos : ArgIn  Port=3  ArgumentName=useRobotPos
  arrived : ArgOut  DisableCoverage=on  OutDataTypeStr=boolean  ArgumentName=arrived
  wires:
  xCoord/1 -> stateflow hasMovedToCoords/1(xCoord)
  yCoord/1 -> stateflow hasMovedToCoords/2(yCoord)
  stateflow hasMovedToCoords/1(hasArrived) -> arrived/1
  useRobotPos/1 -> stateflow hasMovedToCoords/3(useRobotPos)

== system AutonomousModel_V5/function hasSurveyedSides ==
  hasSurveyedSides : TriggerPort  TriggerType=function-call  IsSimulinkFunction=on  FunctionName=hasSurveyedSides  FunctionVisibility=scoped  VariantControl=(inherit)
  function getSurveyAngles : MATLAB Function  TreatAsAtomicUnit=on
  stateflow hasSurveyedSides : Stateflow chart  TreatAsAtomicUnit=on
  pivotSide : ArgIn  DisableCoverage=on  ArgumentName=pivotSide
  sidesSurveyed : ArgOut  DisableCoverage=on  OutDataTypeStr=boolean  ArgumentName=sidesSurveyed
  wires:
  function getSurveyAngles/3(returnAngle) -> stateflow hasSurveyedSides/3(returnAngle)
  stateflow hasSurveyedSides/1(hasSurveyedSides) -> sidesSurveyed/1
  function getSurveyAngles/2(secondSurveyAngle) -> stateflow hasSurveyedSides/2(secondSurveyAngle)
  pivotSide/1 -> function getSurveyAngles/1(pivotSide)
  function getSurveyAngles/1(firstSurveyAngle) -> stateflow hasSurveyedSides/1(firstSurveyAngle)

== system AutonomousModel_V5/function hasTurnedToAngle ==
  note: targetAngle should be from 0 to 360 degrees
  note: PID_SETTLE_TIME is measured in n*0.1 seconds,
      | meaning a value of 5 for this would mean a
      | requirement for the PID to turn the robot should
      | settle for 0.5 seconds before stopping
  hasTurnedToAngle : TriggerPort  TriggerType=function-call  IsSimulinkFunction=on  FunctionName=hasTurnedToAngle  FunctionVisibility=scoped  VariantControl=(inherit)
  Abs : Abs
  Data Store Memory2 : DataStoreMemory  DataStoreName=settledTime  ReadBeforeWriteMsg=warning  WriteAfterWriteMsg=warning  WriteAfterReadMsg=warning  ShowAdditionalParam=off  OutDataTypeStr=double  Dimensions=1
  Data Store Read2 : DataStoreRead  DataStoreName=settledTime
  Data Store Write4 : DataStoreWrite  DataStoreName=leftMotor
  Data Store Write5 : DataStoreWrite  DataStoreName=rightMotor
  Gain : Gain  Gain=-1
  GreaterThanOrEqual : RelationalOperator  OutDataTypeStr=boolean  RndMeth=Simplest
  PID Controller1 : pid_lib/PID Controller  Controller=PI  Form=Parallel  TimeDomain=Discrete-time  UseExternalTs=off  SampleTime=-1  IntegratorMethod=Forward Euler  FilterMethod=Forward Euler  ControllerParametersSource=internal  P=0.812779127376154  I=0  D=0  UseFilter=off  N=100  TunerSelectOption=Transfer Function Based (PID Tuner App)  InitialConditionSource=internal  InitialConditionForIntegrator=0.21807542656823095  InitialConditionForFilter=0  DifferentiatorICPrevScaledInput=0  ExternalReset=none  TrackingMode=off  Kt=1  LimitOutput=on  SatLimitsSource=internal  UpperSaturationLimit=127  LowerSaturationLimit=-127  LinearizeAsGain=off  AntiWindupMode=none  Kb=1  RndMeth=Nearest  POutMin=[]  POutMax=[]  IOutMin=[]  IOutMax=[]  DOutMin=[]  DOutMax=[]  NOutMin=[]  NOutMax=[]  SumOutMin=[]  SumOutMax=[]  SaturationOutMin=[]  SaturationOutMax=[]  PParamMin=[]  PParamMax=[]  IParamMin=[]  IParamMax=[]  DParamMin=[]  DParamMax=[]  NParamMin=[]  NParamMax=[]  KbParamMin=[]  KbParamMax=[]  KtParamMin=[]  KtParamMax=[]  KbOutMin=[]  KbOutMax=[]  KtOutMin=[]  KtOutMax=[]  IntegratorOutMin=[]  IntegratorOutMax=[]  FilterOutMin=[]  FilterOutMax=[]  SumI1OutMin=[]  SumI1OutMax=[]  SumI2OutMin=[]  SumI2OutMax=[]  SumI3OutMin=[]  SumI3OutMax=[]  SumI4OutMin=[]  SumI4OutMax=[]  SumDOutMin=[]  SumDOutMax=[]  DifferentiatorOutMin=[]  DifferentiatorOutMax=[]  FilterDiffOutCoefMin=[]  FilterDiffOutCoefMax=[]  ReciprocalOutMin=[]  ReciprocalOutMax=[]  SumDenOutMin=[]  SumDenOutMax=[]  SumNumOutMin=[]  SumNumOutMax=[]  DivideOutMin=[]  DivideOutMax=[]  UdiffTsProdOutMin=[]  UdiffTsProdOutMax=[]  NTsProdOutMin=[]  NTsProdOutMax=[]  UintegralTsProdOutMin=[]  UintegralTsProdOutMax=[]  UngainTsProdOutMin=[]  UngainTsProdOutMax=[]  IntegratorContinuousStateAttributes=''  IntegratorStateMustResolveToSignalObject=off  IntegratorRTWStateStorageClass=Auto  FilterContinuousStateAttributes=''  FilterStateMustResolveToSignalObject=off  FilterRTWStateStorageClass=Auto  ParallelPVariant=InternalParameters  IdealPVariant=Disabled  IVariant=InternalParameters  DVariant=Disabled  IntegratorVariant=Discrete  SatVariant=Enabled  AWVariant=Passthrough  PCopyVariant=Disabled  TRVariant=Disabled  FdbkBlocksVariant=Forward  IdealPFdbkVariant=Disabled  SatFdbkVariant=Disabled  DerivativeFilterVariant=Disabled  NVariant=Disabled  NCopyVariant=Disabled_SignalSpec  FilterICVariant=Disabled  IntegratorICVariant=InternalICs  ExternalResetVariant=Disabled  TRSumVariant=Passthrough  SumFdbkVariant=Disabled  SumVariant=Sum_PI  TsampFilterVariant=InternalTs  TsampNgainVariant=Passthrough  TsampIntegralVariant=Passthrough  ExternalSaturationOutDataTypeStr=Inherit: Same as second input
  PID Controller2 : pid_lib/PID Controller  Commented=on  Controller=PI  Form=Parallel  TimeDomain=Discrete-time  UseExternalTs=off  SampleTime=-1  IntegratorMethod=Forward Euler  FilterMethod=Forward Euler  ControllerParametersSource=internal  P=0.4220988064561398  I=245.15019805202533  D=0  UseFilter=off  N=100  TunerSelectOption=Transfer Function Based (PID Tuner App)  InitialConditionSource=internal  InitialConditionForIntegrator=0  InitialConditionForFilter=0  DifferentiatorICPrevScaledInput=0  ExternalReset=rising  TrackingMode=off  Kt=1  LimitOutput=on  SatLimitsSource=internal  UpperSaturationLimit=127  LowerSaturationLimit=-127  LinearizeAsGain=off  AntiWindupMode=none  Kb=1  RndMeth=Nearest  POutMin=[]  POutMax=[]  IOutMin=[]  IOutMax=[]  DOutMin=[]  DOutMax=[]  NOutMin=[]  NOutMax=[]  SumOutMin=[]  SumOutMax=[]  SaturationOutMin=[]  SaturationOutMax=[]  PParamMin=[]  PParamMax=[]  IParamMin=[]  IParamMax=[]  DParamMin=[]  DParamMax=[]  NParamMin=[]  NParamMax=[]  KbParamMin=[]  KbParamMax=[]  KtParamMin=[]  KtParamMax=[]  KbOutMin=[]  KbOutMax=[]  KtOutMin=[]  KtOutMax=[]  IntegratorOutMin=[]  IntegratorOutMax=[]  FilterOutMin=[]  FilterOutMax=[]  SumI1OutMin=[]  SumI1OutMax=[]  SumI2OutMin=[]  SumI2OutMax=[]  SumI3OutMin=[]  SumI3OutMax=[]  SumI4OutMin=[]  SumI4OutMax=[]  SumDOutMin=[]  SumDOutMax=[]  DifferentiatorOutMin=[]  DifferentiatorOutMax=[]  FilterDiffOutCoefMin=[]  FilterDiffOutCoefMax=[]  ReciprocalOutMin=[]  ReciprocalOutMax=[]  SumDenOutMin=[]  SumDenOutMax=[]  SumNumOutMin=[]  SumNumOutMax=[]  DivideOutMin=[]  DivideOutMax=[]  UdiffTsProdOutMin=[]  UdiffTsProdOutMax=[]  NTsProdOutMin=[]  NTsProdOutMax=[]  UintegralTsProdOutMin=[]  UintegralTsProdOutMax=[]  UngainTsProdOutMin=[]  UngainTsProdOutMax=[]  IntegratorContinuousStateAttributes=''  IntegratorStateMustResolveToSignalObject=off  IntegratorRTWStateStorageClass=Auto  FilterContinuousStateAttributes=''  FilterStateMustResolveToSignalObject=off  FilterRTWStateStorageClass=Auto  ParallelPVariant=InternalParameters  IdealPVariant=Disabled  IVariant=InternalParameters  DVariant=Disabled  IntegratorVariant=Discrete  SatVariant=Enabled  AWVariant=Passthrough  PCopyVariant=Disabled  TRVariant=Disabled  FdbkBlocksVariant=Forward  IdealPFdbkVariant=Disabled  SatFdbkVariant=Disabled  DerivativeFilterVariant=Disabled  NVariant=Disabled  NCopyVariant=Disabled_SignalSpec  FilterICVariant=Disabled  IntegratorICVariant=InternalICs  ExternalResetVariant=ExternalReset  TRSumVariant=Passthrough  SumFdbkVariant=Disabled  SumVariant=Sum_PI  TsampFilterVariant=InternalTs  TsampNgainVariant=Passthrough  TsampIntegralVariant=Passthrough  ExternalSaturationOutDataTypeStr=Inherit: Same as second input
  PID_ANGLE_TOLERANCE : Constant  Value=0.3
  PID_SETTLE_TIME : Constant  Value=0.5
  function fixUserAngle : MATLAB Function  TreatAsAtomicUnit=on
  stateflow integrateSettleTime : Stateflow chart  TreatAsAtomicUnit=on
      settings: PortSchema="{\"entries\":[{\"content\":{\"sides\":[{\"content\":{\"connectorIds\":[\"In2\",\"In1\"]},\"type\":\"ConnectorPlacement.EquallySpacedRectSide\",\"uuid\":\"f923337d-3128-4ed8-bb4f-3ea7b5686e2d\"},{\"content\":{\"connectorIds\":[],\"side\":\"RIGHT\"},\"type\":\"ConnectorPlacement.EquallySpacedRectSide\",\"uuid\":\"39dc7172-a5aa-4f5c-b2a4-4c61f2fa72eb\"},{\"content\":{\"connectorIds\":[],\"side\":\"TOP\"},\"type\":\"ConnectorPlacement.EquallySpacedRectSide\",\"uuid\":\"39425eec-6ca1-4a0a-a982-d9b02b3e3e8f\"},{\"content\":{\"connectorIds\":[],\"side\":\"HIDDEN\"},\"type\":\"ConnectorPlacement.EquallySpacedRectSide\",\"uuid\":\"aee45ecb-1b8b-4c38-bfd6-fdbe8fac54d7\"}]},\"type\":\"ConnectorPlacement.EquallySpacedConnector\",\"uuid\":\"e05cbbda-f452-42ce-8e08-9c45c77a95c5\"}],\"packageUris\":[\"http://schema.mathworks.com/mf0/Connector/R2020b\"],\"version\":\"1.0\"}"
  stateflow postSettleAngle : Stateflow chart  TreatAsAtomicUnit=on
  targetAngle : ArgIn  DisableCoverage=on  ArgumentName=targetAngle
  angleHasSettled : ArgOut  DisableCoverage=on  OutDataTypeStr=boolean  ArgumentName=angleHasSettled
  wires:
  GreaterThanOrEqual/1 -> stateflow postSettleAngle/1(angleHasSettled), angleHasSettled/1
  targetAngle/1 -> function fixUserAngle/1(targetAngle)
  Data Store Read2/1 -> GreaterThanOrEqual/1
  Gain/1 -> Data Store Write4/1
  PID_ANGLE_TOLERANCE/1 -> stateflow integrateSettleTime/1(TOLERANCE)
  PID_SETTLE_TIME/1 -> GreaterThanOrEqual/2
  Abs/1 -> stateflow integrateSettleTime/2(error)
  PID Controller1/1 -> Gain/1, Data Store Write5/1
  function fixUserAngle/1(optimalAngleDiff) -> Abs/1, PID Controller1/1

== system AutonomousModel_V5/function surveySweepHasFoundCell ==
  surveySweepHasFoundCell : TriggerPort  TriggerType=function-call  IsSimulinkFunction=on  FunctionName=surveySweepHasFoundCell  FunctionVisibility=scoped  VariantControl=(inherit)
  function cellCriteriaFound : Subsystem  TreatAsAtomicUnit=on
  stateflow surveySweepHasFoundCell : Stateflow chart  TreatAsAtomicUnit=on
  gridX : ArgIn  ArgumentName=gridX
  gridY : ArgIn  Port=2  ArgumentName=gridY
  onlyUninfected : ArgIn  Port=3  OutDataTypeStr=boolean  ArgumentName=onlyUninfected
  cellFound : ArgOut  OutDataTypeStr=boolean  ArgumentName=cellFound
  wires:
  stateflow surveySweepHasFoundCell/1(cellFound) -> cellFound/1
  gridX/1 -> stateflow surveySweepHasFoundCell/1(gridX)
  gridY/1 -> stateflow surveySweepHasFoundCell/2(gridY)
  onlyUninfected/1 -> stateflow surveySweepHasFoundCell/3(onlyUninfected)

== system AutonomousModel_V5/stateflow MAIN_PROGRAM/MAIN_PROGRAM.hasClearedPlatformAt ==
  gridX : Inport  OutDataTypeStr=double  PortDimensions=1
  gridY : Inport  Port=2  OutDataTypeStr=double  PortDimensions=1
  f : TriggerPort  TriggerType=function-call  VariantControl=(inherit)
      settings: CopyFcn=Stateflow.SLINSF.SimulinkMan.removeBlockPreDeleteFcn  PreDeleteFcn=Stateflow.SLINSF.SimulinkMan.unsafePredeleteFcn
  stateflow hasClearedPlatformAt : Stateflow chart  TreatAsAtomicUnit=on
  platformCleared : Outport
  wires:
  stateflow hasClearedPlatformAt/1(platformCleared) -> platformCleared/1
  gridX/1 -> stateflow hasClearedPlatformAt/1(gridX)
  gridY/1 -> stateflow hasClearedPlatformAt/2(gridY)

== system AutonomousModel_V5/stateflow MAIN_PROGRAM/MAIN_PROGRAM.hasDroppedVacAt ==
  xCoord : Inport  OutDataTypeStr=double  PortDimensions=1
  yCoord : Inport  Port=2  OutDataTypeStr=double  PortDimensions=1
  f : TriggerPort  TriggerType=function-call  VariantControl=(inherit)
      settings: CopyFcn=Stateflow.SLINSF.SimulinkMan.removeBlockPreDeleteFcn  PreDeleteFcn=Stateflow.SLINSF.SimulinkMan.unsafePredeleteFcn
  Stateflow : Stateflow chart  TreatAsAtomicUnit=on
  function dropVaccine : Subsystem  TreatAsAtomicUnit=on
  deliveredVac : Outport
  wires:
  xCoord/1 -> Stateflow/1(xCoord)
  yCoord/1 -> Stateflow/2(yCoord)
  Stateflow/1(vaccineDropped) -> deliveredVac/1

== system AutonomousModel_V5/stateflow MAIN_PROGRAM/MAIN_PROGRAM.hasSavedAllUninfected ==
  f : TriggerPort  TriggerType=function-call  VariantControl=(inherit)
      settings: CopyFcn=Stateflow.SLINSF.SimulinkMan.removeBlockPreDeleteFcn  PreDeleteFcn=Stateflow.SLINSF.SimulinkMan.unsafePredeleteFcn
  stateflow hasSavedAllUninfected : Stateflow chart  TreatAsAtomicUnit=on
  allUninfectedSaved : Outport
  wires:
  stateflow hasSavedAllUninfected/1(allUninfectedSaved) -> allUninfectedSaved/1
